simulink model "pyramid_sim"  (R2019a)
settings: Solver=VariableStepAuto  StartTime=0.0  StopTime=30  RelTol=1e-3
values from neighbouring files (symbols this model uses):
  inertia = eye(3)    [simulation.m]
  K = eye(6)*25    [simulation.m]
  Sig = eye(6)    [simulation.m]
libraries: simulink x2, shared6dof x1, sharedtransform x1
settings Model: Creator=marin  LastModifiedBy=marin
settings SolverCC: ZeroCrossAlgorithm=Adaptive
settings DebuggingCC: IgnoredZcDiagnostic=none

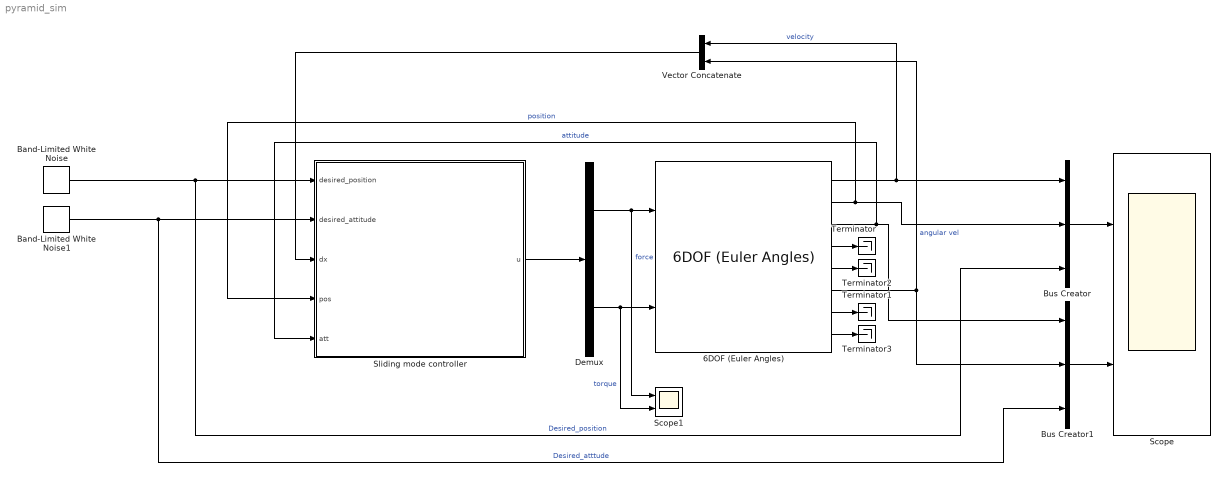
== system pyramid_sim ==
  6DOF (Euler Angles) : shared6dof/6DOF (Euler Angles)  units=Metric (MKS)  mtype=Fixed  rep=Euler Angles  xme_0=[0 0 0]  Vm_0=[0 0 0]  eul_0=[0 0 0]  pm_0=[0 0 0]  mass_0=1.0  mass_e=0.5  mass_f=2.0  inertia=eye(3)  inertia_e=eye(3)  inertia_f=2*eye(3)  k_quat=1.0  vre_flag=on  abi_flag=off  aMode=0  xme_statename=''  Vm_statename=''  eul_statename=''  quat_statename=''  pm_statename=''  mass_statename=''
      settings: SourceProductBaseCode=AE
  Band-Limited White Noise : simulink/Sources/Band-Limited White Noise  Cov=[0.7, 1.1, 0.3]'  Ts=3  seed=[23, 3, 41]'
  Band-Limited White Noise1 : simulink/Sources/Band-Limited White Noise  Cov=[1.4, 1.3, 1.7]'  Ts=3  seed=[123, 113, 4111]'
  Bus Creator : BusCreator  Inputs=3
  Bus Creator1 : BusCreator  Inputs=3
  Demux : Demux  Outputs=2
  Scope : Scope  NumInputPorts=2
  Scope1 : Scope  NumInputPorts=2
  Sliding mode controller : Subsystem
  Terminator{,1..3} (4 alike) : Terminator
  Vector Concatenate : Concatenate
  wires:
  Demux/2 -> Scope1/2, 6DOF (Euler Angles)/2  "torque"
  Demux/1 -> Scope1/1, 6DOF (Euler Angles)/1  "force"
  Sliding mode controller/1(u) -> Demux/1
  6DOF (Euler Angles)/1 -> Bus Creator/1, Vector Concatenate/1  "velocity"
  6DOF (Euler Angles)/6 -> Bus Creator1/2, Vector Concatenate/2  "angular vel"
  6DOF (Euler Angles)/2 -> Bus Creator/2, Sliding mode controller/4(pos)  "position"
  Vector Concatenate/1 -> Sliding mode controller/3(dx)
  Band-Limited White Noise1/1 -> Bus Creator1/3, Sliding mode controller/2(desired_attitude)  "Desired_atttude"
  Band-Limited White Noise/1 -> Bus Creator/3, Sliding mode controller/1("desired_position ")  "Desired_position"
  6DOF (Euler Angles)/3 -> Bus Creator1/1, Sliding mode controller/5(att)  "attitude"
  6DOF (Euler Angles)/4 -> Terminator/1
  6DOF (Euler Angles)/7 -> Terminator1/1
  6DOF (Euler Angles)/5 -> Terminator2/1
  6DOF (Euler Angles)/8 -> Terminator3/1
  Bus Creator1/1 -> Scope/2
  Bus Creator/1 -> Scope/1

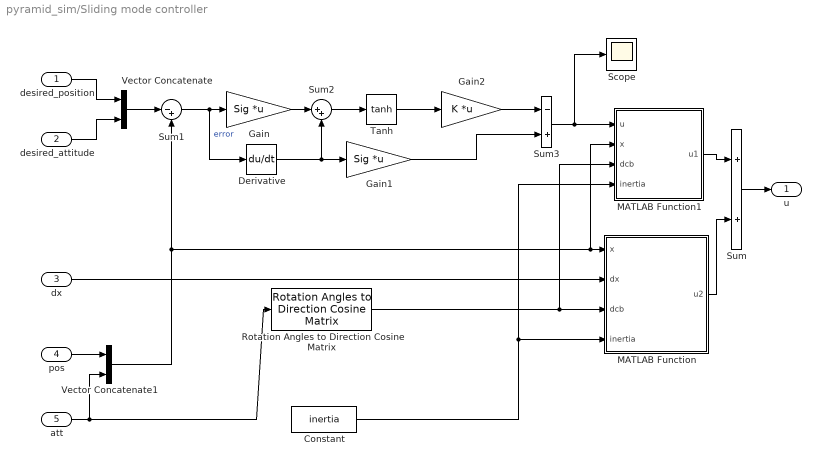
== system pyramid_sim/Sliding mode controller ==
  "desired_position " : Inport
  desired_attitude : Inport  Port=2
  dx : Inport  Port=3
  pos : Inport  Port=4
  att : Inport  Port=5
  Constant : Constant  Value=inertia
  Derivative : Derivative
  Gain : Gain  Gain=Sig  Multiplication=Matrix(K*u) (u vector)
  Gain1 : Gain  Gain=Sig  Multiplication=Matrix(K*u) (u vector)
  Gain2 : Gain  Gain=K  Multiplication=Matrix(K*u) (u vector)
  MATLAB Function : MATLAB Function  TreatAsAtomicUnit=on
  MATLAB Function1 : MATLAB Function  TreatAsAtomicUnit=on
  Rotation Angles to Direction Cosine Matrix : sharedtransform/Rotation Angles to Direction Cosine Matrix  rotationOrder=ZYX  aMode=aMode
      settings: SourceProductBaseCode=AE
  Scope : Scope
  Sum : Sum
  Sum1 : Sum  Inputs=|-+
  Sum2 : Sum  Inputs=|++
  Sum3 : Sum  Inputs=-+
  Tanh : Trigonometry  Operator=tanh
  Vector Concatenate : Concatenate
  Vector Concatenate1 : Concatenate
  u : Outport
  wires:
  Sum/1 -> u/1
  desired_attitude/1 -> Vector Concatenate/2
  "desired_position "/1 -> Vector Concatenate/1
  Vector Concatenate/1 -> Sum1/1
  Sum1/1 -> Derivative/1, Gain/1  "error"
  Gain/1 -> Sum2/1
  Derivative/1 -> Gain1/1, Sum2/2
  Gain1/1 -> Sum3/2
  Tanh/1 -> Gain2/1
  Gain2/1 -> Sum3/1
  Vector Concatenate1/1 -> MATLAB Function1/2(x), MATLAB Function/1(x), Sum1/2
  dx/1 -> MATLAB Function/2(dx)
  Rotation Angles to Direction Cosine Matrix/1 -> MATLAB Function/3(dcb), MATLAB Function1/3(dcb)
  MATLAB Function/1(u2) -> Sum/2
  Sum3/1 -> Scope/1, MATLAB Function1/1(u)
  MATLAB Function1/1(u1) -> Sum/1
  Constant/1 -> MATLAB Function/4(inertia), MATLAB Function1/4(inertia)
  pos/1 -> Vector Concatenate1/1
  att/1 -> Vector Concatenate1/2, Rotation Angles to Direction Cosine Matrix/1
  Sum2/1 -> Tanh/1

== matlab function pyramid_sim/Sliding mode controller/MATLAB Function1 ==
  data: u input; x input; u1 output; dcb input; inertia input
function u1 = Minvx(u, x, dcb, inertia)

Ig = dcb'*inertia*dcb;

%S = zeros(3, 3);
S = [1,          0,          -sin(x(5));
     0,  cos(x(4)), cos(x(5))*sin(x(4));
     0, -sin(x(4)), cos(x(5))*cos(x(4));];

M = zeros(6, 6);
M(1:3, 1:3) = eye(3);
M(4:6, 4:6) = S'*Ig*S;

u1 = M \ u;

== matlab function pyramid_sim/Sliding mode controller/MATLAB Function ==
  data: x input; u2 output; dx input; dcb input; inertia input
function u2 = model(x, dx, dcb, inertia)

Ig = dcb'*inertia*dcb;

%S = zeros(3, 3);
S = [1,          0,          -sin(x(5));
     0,  cos(x(4)), cos(x(5))*sin(x(4));
     0, -sin(x(4)), cos(x(5))*cos(x(4));];

%dS = zeros(3, 3);
dS = [0,          0,                                 -cos(x(5));
      0, -sin(x(4)), -sin(x(5))*sin(x(4)) + cos(x(5))*cos(x(4));
      0, -cos(x(4)), -sin(x(5))*cos(x(4)) - cos(x(5))*sin(x(4));];
  
skew = [     0, -dx(6),  dx(5);
        -dx(6),      0, -dx(4);
        -dx(5),  dx(4),      0;];
 
C = zeros(6, 6);
C(4:6, 4:6) = S'*Ig*dS + S'*skew*Ig*S;
 
u2 = C*dx;
